simulink model "controller_framework_static_decoupled"  (R2016a)
settings: Solver=VariableStepAuto  StartTime=0.0  StopTime=800  RelTol=1e-3
libraries: simulink x2
settings Model: Creator=mikae  LastModifiedBy=jamie

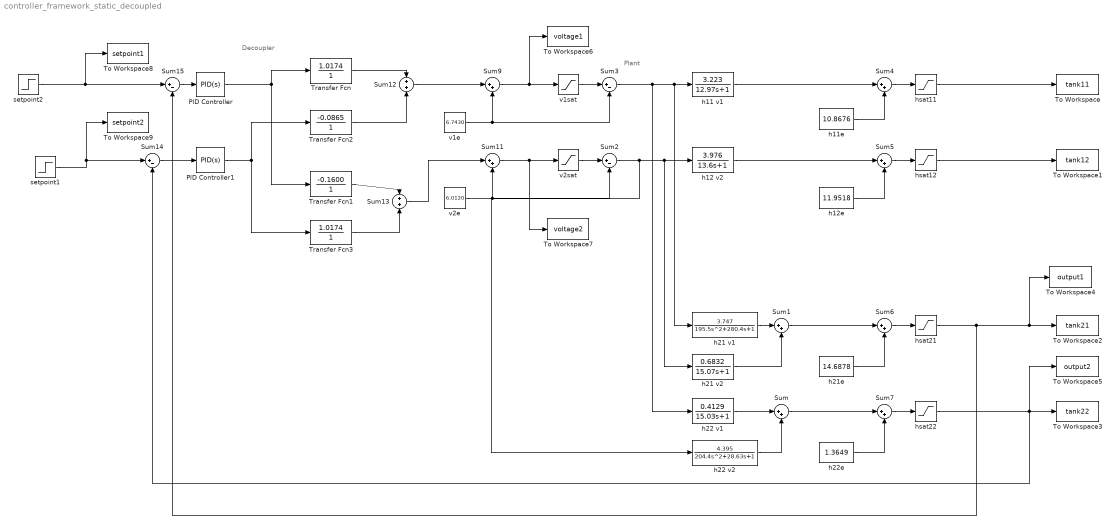
== system controller_framework_static_decoupled ==
  note: Decoupler
  note: Plant
  PID Controller : simulink/Continuous/PID Controller  Controller=PID  TimeDomain=Continuous-time  SampleTime=-1  IntegratorMethod=Forward Euler  FilterMethod=Forward Euler  Form=Parallel  UseFilter=on  ControllerParametersSource=internal  P=1.4351  I=0.0051437  D=10.0105  N=100  InitialConditionSource=internal  InitialConditionForIntegrator=0  InitialConditionForFilter=0  ExternalReset=none  LimitOutput=off  UpperSaturationLimit=inf  LowerSaturationLimit=-inf  LinearizeAsGain=on  AntiWindupMode=none  Kb=1  TrackingMode=off  Kt=1  PParamMin=[]  PParamMax=[]  IParamMin=[]  IParamMax=[]  DParamMin=[]  DParamMax=[]  NParamMin=[]  NParamMax=[]  KbParamMin=[]  KbParamMax=[]  KtParamMin=[]  KtParamMax=[]  POutMin=[]  POutMax=[]  IOutMin=[]  IOutMax=[]  DOutMin=[]  DOutMax=[]  NOutMin=[]  NOutMax=[]  KbOutMin=[]  KbOutMax=[]  KtOutMin=[]  KtOutMax=[]  IntegratorOutMin=[]  IntegratorOutMax=[]  FilterOutMin=[]  FilterOutMax=[]  SumOutMin=[]  SumOutMax=[]  SumI1OutMin=[]  SumI1OutMax=[]  SumI2OutMin=[]  SumI2OutMax=[]  SumI3OutMin=[]  SumI3OutMax=[]  SumDOutMin=[]  SumDOutMax=[]  SaturationOutMin=[]  SaturationOutMax=[]  IntegratorContinuousStateAttributes=''  IntegratorStateMustResolveToSignalObject=off  IntegratorRTWStateStorageClass=Auto  FilterContinuousStateAttributes=''  FilterStateMustResolveToSignalObject=off  FilterRTWStateStorageClass=Auto  DifferentiatorICPrevScaledInput=0  DifferentiatorOutMin=[]  DifferentiatorOutMax=[]
  PID Controller1 : simulink/Continuous/PID Controller  Controller=PID  TimeDomain=Continuous-time  SampleTime=-1  IntegratorMethod=Forward Euler  FilterMethod=Forward Euler  Form=Parallel  UseFilter=on  ControllerParametersSource=internal  P=1.4351  I=0.0051437  D=10.0105  N=100  InitialConditionSource=internal  InitialConditionForIntegrator=0  InitialConditionForFilter=0  ExternalReset=none  LimitOutput=off  UpperSaturationLimit=inf  LowerSaturationLimit=-inf  LinearizeAsGain=on  AntiWindupMode=none  Kb=1  TrackingMode=off  Kt=1  PParamMin=[]  PParamMax=[]  IParamMin=[]  IParamMax=[]  DParamMin=[]  DParamMax=[]  NParamMin=[]  NParamMax=[]  KbParamMin=[]  KbParamMax=[]  KtParamMin=[]  KtParamMax=[]  POutMin=[]  POutMax=[]  IOutMin=[]  IOutMax=[]  DOutMin=[]  DOutMax=[]  NOutMin=[]  NOutMax=[]  KbOutMin=[]  KbOutMax=[]  KtOutMin=[]  KtOutMax=[]  IntegratorOutMin=[]  IntegratorOutMax=[]  FilterOutMin=[]  FilterOutMax=[]  SumOutMin=[]  SumOutMax=[]  SumI1OutMin=[]  SumI1OutMax=[]  SumI2OutMin=[]  SumI2OutMax=[]  SumI3OutMin=[]  SumI3OutMax=[]  SumDOutMin=[]  SumDOutMax=[]  SaturationOutMin=[]  SaturationOutMax=[]  IntegratorContinuousStateAttributes=''  IntegratorStateMustResolveToSignalObject=off  IntegratorRTWStateStorageClass=Auto  FilterContinuousStateAttributes=''  FilterStateMustResolveToSignalObject=off  FilterRTWStateStorageClass=Auto  DifferentiatorICPrevScaledInput=0  DifferentiatorOutMin=[]  DifferentiatorOutMax=[]
  Sum{,1,4..7,9,11} (8 alike) : Sum  Inputs=|++
  Sum12 : Sum
  Sum13 : Sum
  Sum{2..3,14..15} (4 alike) : Sum  Inputs=|+-
  To Workspace : ToWorkspace  VariableName=tank11  SaveFormat=Timeseries  SampleTime=-1
  To Workspace1 : ToWorkspace  VariableName=tank12  SaveFormat=Timeseries  SampleTime=-1
  To Workspace2 : ToWorkspace  VariableName=tank21  SaveFormat=Timeseries  SampleTime=-1
  To Workspace3 : ToWorkspace  VariableName=tank22  SaveFormat=Timeseries  SampleTime=-1
  To Workspace4 : ToWorkspace  VariableName=output1  SaveFormat=Timeseries  SampleTime=-1
  To Workspace5 : ToWorkspace  VariableName=output2  SaveFormat=Timeseries  SampleTime=-1
  To Workspace6 : ToWorkspace  VariableName=voltage1  SaveFormat=Timeseries  SampleTime=-1
  To Workspace7 : ToWorkspace  VariableName=voltage2  SaveFormat=Timeseries  SampleTime=-1
  To Workspace8 : ToWorkspace  VariableName=setpoint1  SaveFormat=Timeseries  SampleTime=-1
  To Workspace9 : ToWorkspace  VariableName=setpoint2  SaveFormat=Timeseries  SampleTime=-1
  Transfer Fcn : TransferFcn  Numerator=[1.0174]  Denominator=[1]
  Transfer Fcn1 : TransferFcn  Numerator=[-0.1600]  Denominator=[1]
  Transfer Fcn2 : TransferFcn  Numerator=[-0.0865]  Denominator=[1]
  Transfer Fcn3 : TransferFcn  Numerator=[1.0174]  Denominator=[1]
  h11 v1 : TransferFcn  Numerator=[3.223]  Denominator=[12.97 1]
  h11e : Constant  Value=10.8676
  h12 v2 : TransferFcn  Numerator=[3.976]  Denominator=[13.6 1]
  h12e : Constant  Value=11.9518
  h21 v1 : TransferFcn  Numerator=[3.747]  Denominator=[195.5 280.4 1]
  h21 v2 : TransferFcn  Numerator=[0.6832]  Denominator=[15.07 1]
  h21e : Constant  Value=14.6878
  h22 v1 : TransferFcn  Numerator=[0.4129]  Denominator=[15.03 1]
  h22 v2 : TransferFcn  Numerator=[4.395]  Denominator=[204.4 28.63 1]
  h22e : Constant  Value=1.3649
  hsat{11..12,21..22} (4 alike) : Saturate  UpperLimit=30  LowerLimit=0
  setpoint1 : Step  Time=30  Before=22.5  After=26.55  SampleTime=0
  setpoint2 : Step  Before=22.5  After=26.55  SampleTime=0
  v1e : Constant  Value=6.7430
  v1sat : Saturate  UpperLimit=12  LowerLimit=0
  v2e : Constant  Value=6.0120
  v2sat : Saturate  UpperLimit=12  LowerLimit=0
  wires:
  Sum9/1 -> To Workspace6/1, v1sat/1
  h21 v1/1 -> Sum1/1
  h21 v2/1 -> Sum1/2
  h22 v1/1 -> Sum/1
  h22 v2/1 -> Sum/2
  h11 v1/1 -> Sum4/1
  Sum5/1 -> hsat12/1
  h12 v2/1 -> Sum5/1
  Sum1/1 -> Sum6/1
  Sum6/1 -> hsat21/1
  Sum/1 -> Sum7/1
  Sum7/1 -> hsat22/1
  v1sat/1 -> Sum3/1
  v2sat/1 -> Sum2/1
  Sum3/1 -> h22 v1/1, h21 v1/1, h11 v1/1
  Sum2/1 -> h22 v2/1, h21 v2/1, h12 v2/1
  h11e/1 -> Sum4/2
  h12e/1 -> Sum5/2
  h21e/1 -> Sum6/2
  h22e/1 -> Sum7/2
  v1e/1 -> Sum9/2, Sum3/2
  hsat11/1 -> To Workspace/1
  Sum4/1 -> hsat11/1
  PID Controller/1 -> Transfer Fcn/1, Transfer Fcn1/1
  PID Controller1/1 -> Transfer Fcn3/1, Transfer Fcn2/1
  Transfer Fcn3/1 -> Sum13/2
  Transfer Fcn1/1 -> Sum13/1
  Transfer Fcn2/1 -> Sum12/2
  Transfer Fcn/1 -> Sum12/1
  Sum12/1 -> Sum9/1
  Sum11/1 -> To Workspace7/1, v2sat/1
  Sum13/1 -> Sum11/1
  v2e/1 -> Sum11/2, Sum2/2
  hsat12/1 -> To Workspace1/1
  setpoint1/1 -> To Workspace9/1, Sum14/1
  hsat22/1 -> To Workspace3/1, To Workspace5/1, Sum14/2
  setpoint2/1 -> To Workspace8/1, Sum15/1
  hsat21/1 -> To Workspace4/1, To Workspace2/1, Sum15/2
  Sum15/1 -> PID Controller/1
  Sum14/1 -> PID Controller1/1
